simulink model "discrete_PID_anti_windup_3_1_1_b"  (R2024b)
settings: Solver=ode5  StartTime=0.0  StopTime=20  FixedStep=0.001  RelTol=1e-3
undefined symbols (not defined in the file): control_input, DiscIntNeverNeededParam, K_W, kd, ki, kp, National_Instruments, PCI, sens, T, tl, u_bar_max
libraries: sldrtlib x3
settings Model: SimulationMode=external  ExtModeTrigDuration=20001  Creator=fasoloandr  LastModifiedBy=Enrico
settings DataIOCC: ReturnWorkspaceOutputs=off
settings HardwareCC: ProdBitPerLong=64  ProdHWDeviceType=Intel->x86-64 (Linux 64)
settings RTWCC: Description=Simulink Desktop Real-Time  SystemTargetFile=sldrt.tlc  TemplateMakefile=sldrt.tmf  RTWCompilerOptimization=on
settings CodeAppCC: MaxIdLength=95
settings SimulinkDesktopRealTimeCC: TargetLibSuffix=_sldrt.a  TargetPreCompLibLocation=D:\Programmi (D)\MATLAB\R2024b\toolbox\sldrt\lib\win64  ParMdlRefBuildCompliant=on

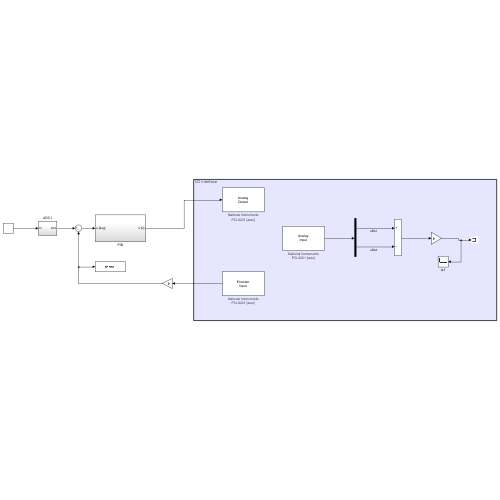
[thumbnail: Simulink's stored preview of the top-level diagram]
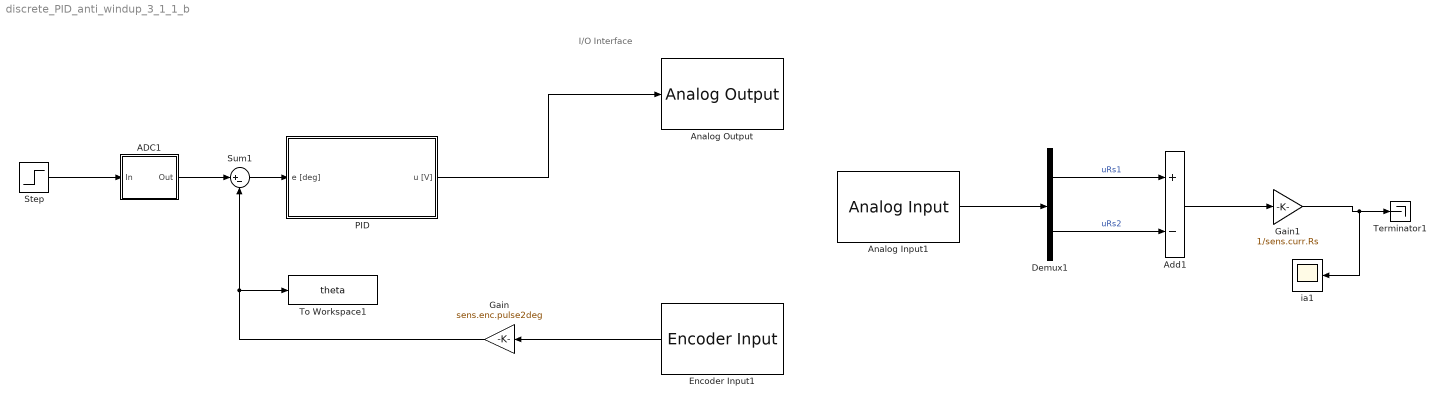
== system discrete_PID_anti_windup_3_1_1_b ==
  note: I/O Interface
  ADC1 : Subsystem
  Add1 : Sum  Inputs=+-
  Analog Input1 : sldrtlib/Analog Input  SampleTime=-1  MaxMissedTicks=10  ShowMissedTicks=off  YieldWhenWaiting=off  DrvName=National_Instruments/PCI-6221  DrvAddress=4294967295  DrvOptions=[0 0 0 2 0]  Channels=[1,2]  RangeMode=1  VoltRange=1  DataType=1
      settings: AttributesFormatString=National Instruments\nPCI-6221 [auto]
  Analog Output : sldrtlib/Analog Output  SampleTime=-1  MaxMissedTicks=10  ShowMissedTicks=off  YieldWhenWaiting=off  DrvName=National_Instruments/PCI-6221  DrvAddress=4294967295  DrvOptions=[0 0 0 2 0]  Channels=1  RangeMode=1  VoltRange=1  InitialValue=[0]  FinalValue=[0]
      settings: AttributesFormatString=National Instruments\nPCI-6221 [auto]
  Demux1 : Demux  Outputs=2
  Encoder Input1 : sldrtlib/Encoder Input  SampleTime=-1  MaxMissedTicks=10  ShowMissedTicks=off  YieldWhenWaiting=off  DrvName=National_Instruments/PCI-6221  DrvAddress=4294967295  DrvOptions=[0 0 0 2 0]  Channels=1  QuadMode=3  IndexPulse=1  InputFilter=Inf  DataType=1
      settings: AttributesFormatString=National Instruments\nPCI-6221 [auto]
  Gain : Gain  Gain=sens.enc.pulse2deg
  Gain1 : Gain  Gain=1/sens.curr.Rs
  PID : Subsystem
  Step : Step  After=360  SampleTime=0
  Sum1 : Sum  Inputs=|+-
  Terminator1 : Terminator
  To Workspace1 : ToWorkspace  VariableName=theta  SaveFormat=Structure With Time  SampleTime=-1
  ia1 : Scope
  wires:
  Gain1/1 -> ia1/1, Terminator1/1
  Demux1/1 -> Add1/1  "uRs1"
  Analog Input1/1 -> Demux1/1
  Demux1/2 -> Add1/2  "uRs2"
  Encoder Input1/1 -> Gain/1
  Add1/1 -> Gain1/1
  Step/1 -> ADC1/1(In)
  ADC1/1(Out) -> Sum1/1
  Gain/1 -> Sum1/2, To Workspace1/1
  Sum1/1 -> PID/1(e [deg])
  PID/1(u [V]) -> Analog Output/1

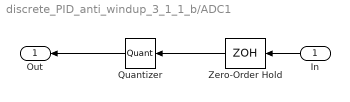
== system discrete_PID_anti_windup_3_1_1_b/ADC1 ==
  In : Inport
  Quantizer : Quantizer  QuantizationInterval=daq.adc.q
  Zero-Order Hold : ZeroOrderHold  SampleTime=T
  Out : Outport
  wires:
  Quantizer/1 -> Out/1
  In/1 -> Zero-Order Hold/1
  Zero-Order Hold/1 -> Quantizer/1

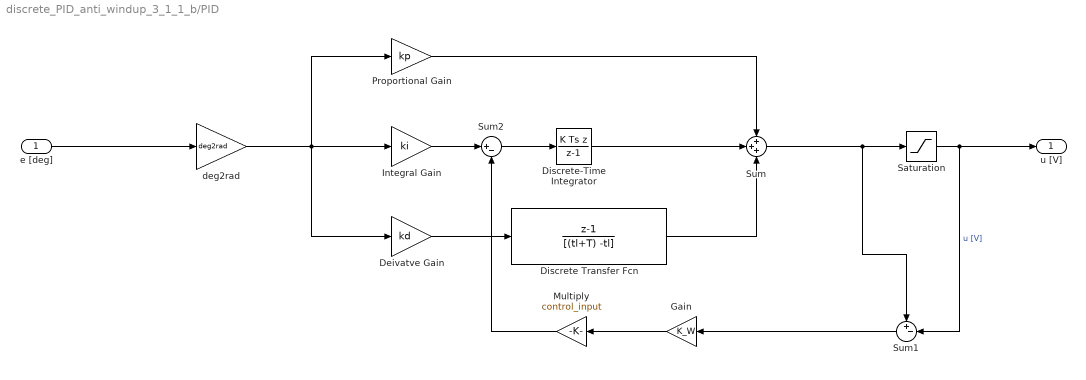
== system discrete_PID_anti_windup_3_1_1_b/PID ==
  e [deg] : Inport
  Deivatve Gain : Gain  Gain=kd
  Discrete Transfer Fcn : DiscreteTransferFcn  Numerator=[1 -1]  Denominator=[(tl+T) -tl]
  Discrete-Time Integrator : DiscreteIntegrator  IntegratorMethod=Integration: Backward Euler  SampleTime=T  ICPrevOutput=DiscIntNeverNeededParam  ICPrevScaledInput=DiscIntNeverNeededParam
  Gain : Gain  Gain=K_W
  Integral Gain : Gain  Gain=ki
  Multiply : Gain  Gain=control_input
  Proportional Gain : Gain  Gain=kp
  "Saturation " : Saturate  UpperLimit=u_bar_max  LowerLimit=-u_bar_max
  Sum : Sum  Inputs=+++
  Sum1 : Sum  Inputs=+-|
  Sum2 : Sum  Inputs=|+-
  deg2rad : Gain  Gain=deg2rad
  u [V] : Outport
  wires:
  Deivatve Gain/1 -> Discrete Transfer Fcn/1
  e [deg]/1 -> deg2rad/1
  "Saturation "/1 -> Sum1/2, u [V]/1  "u [V]"
  deg2rad/1 -> Deivatve Gain/1, Proportional Gain/1, Integral Gain/1
  Discrete Transfer Fcn/1 -> Sum/3
  Proportional Gain/1 -> Sum/1
  Sum/1 -> Sum1/1, "Saturation "/1
  Discrete-Time Integrator/1 -> Sum/2
  Sum1/1 -> Gain/1
  Sum2/1 -> Discrete-Time Integrator/1
  Integral Gain/1 -> Sum2/1
  Gain/1 -> Multiply/1
  Multiply/1 -> Sum2/2
